simulink model "ex1"  (R2024b)
settings: Solver=ode23t  StartTime=0.0  StopTime=5  RelTol=1e-3
libraries: fl_lib x64, nesl_utility x38, ee_lib x30, sdl_lib x8, spsAsynchronousMachineSIUnitsLib x2, spsAsynchronousMachinepuUnitsLib x1
(part 3 of 3)

== system ex1/Erotima_3/Weight6 ==
  Ideal Force Source : fl_lib/Mechanical/Mechanical Sources/Ideal Force Source
  Mass : fl_lib/Mechanical/Translational Elements/Mass  mass=wmass kg  num_ports=foundation.enum.numPorts2.two  v_specify=off  v_priority=High  v=0 m/s  v_nominal_specify=off  v_nominal_value=1  v_nominal_unit=m/s  f_specify=off  f_priority=None  f=0 N  f_nominal_specify=off  f_nominal_value=0  f_nominal_unit=N
      settings: InternalSimscapePortConfiguration="{\"Bottom\":[],\"Left\":[{\"id\":\"M\",\"label\":\"\",\"type\":\"foundation.mechanical.translational.translational\"}],\"Right\":[{\"id\":\"N\",\"label\":\"\",\"type\":\"foundation.mechanical.translational.translational\"}],\"Top\":[]}"
  Mechanical Translational Reference1 : fl_lib/Mechanical/Translational Elements/Mechanical Translational Reference
  Weight : fl_lib/Physical Signals/Sources/PS Constant  constant=-wmass * 9.81
  W : PMIOPort  Side=Right
  connections:
  W/RConn1 -- Mass/LConn1
  Mass/RConn1 -- Ideal Force Source/LConn1
  Mechanical Translational Reference1/LConn1 -- Ideal Force Source/RConn2
  Weight/RConn1 -- Ideal Force Source/RConn1
